simulink model "SimulinkEspacodeEstados"  (R2023a)
settings: Solver=VariableStepAuto  StartTime=0.0  StopTime=10.0  RelTol=1e-3
values from neighbouring files (symbols this model uses):
  A = [0 1; -K/M -b/M]    [ProjetoEspacoEstadosExemplo.m]    (also in ProjetoStateSpace.m = [-1 3; -2 -3])
  B = [0; 1/M]    [ProjetoEspacoEstadosExemplo.m]    (also in ProjetoStateSpace.m = [0; 5])
  kras = [double(kras.k1(1)) double(kras.k2(1)) double(kras.h1(1))]    [ProjetoStateSpace.m]
settings Model: Creator=a2270340  LastModifiedBy=a2270340

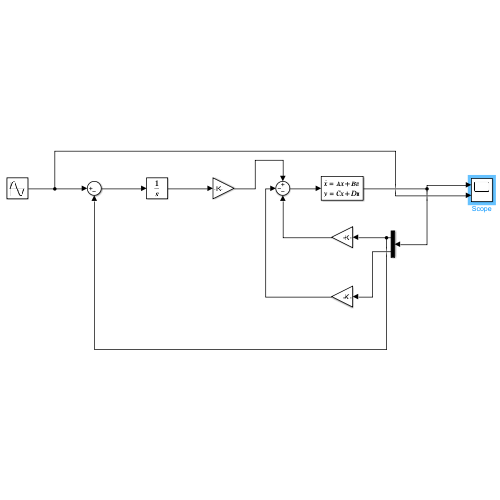
[thumbnail: Simulink's stored preview of the top-level diagram]
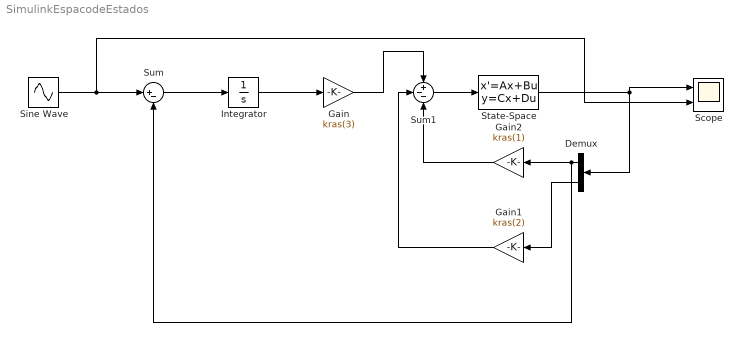
== system SimulinkEspacodeEstados ==
  Demux : Demux  Outputs=2
  Gain : Gain  Gain=kras(3)
  Gain1 : Gain  Gain=kras(2)
  Gain2 : Gain  Gain=kras(1)
  Integrator : Integrator
  Scope : Scope  NumInputPorts=2
  Sine Wave : Sin  Amplitude=500  SampleTime=0
  State-Space : StateSpace  A=A  B=B  C=[1 0; 0 1]  D=[0;0]  InitialCondition=0
  Sum : Sum  Inputs=|+-
  Sum1 : Sum  Inputs=+--
  wires:
  Sum1/1 -> State-Space/1
  Gain/1 -> Sum1/1
  Integrator/1 -> Gain/1
  Sum/1 -> Integrator/1
  Gain2/1 -> Sum1/3
  Gain1/1 -> Sum1/2
  Sine Wave/1 -> Scope/2, Sum/1
  Demux/1 -> Gain2/1, Sum/2
  State-Space/1 -> Demux/1, Scope/1
  Demux/2 -> Gain1/1
